simulink subsystem "OGBMS"  (R2020b)
settings: Solver=VariableStepAuto  StartTime=0.0  StopTime=10.0  RelTol=1e-3
libraries: fl_lib x26, nesl_utility x14
settings Model: Creator=marti  LastModifiedBy=MSI PC

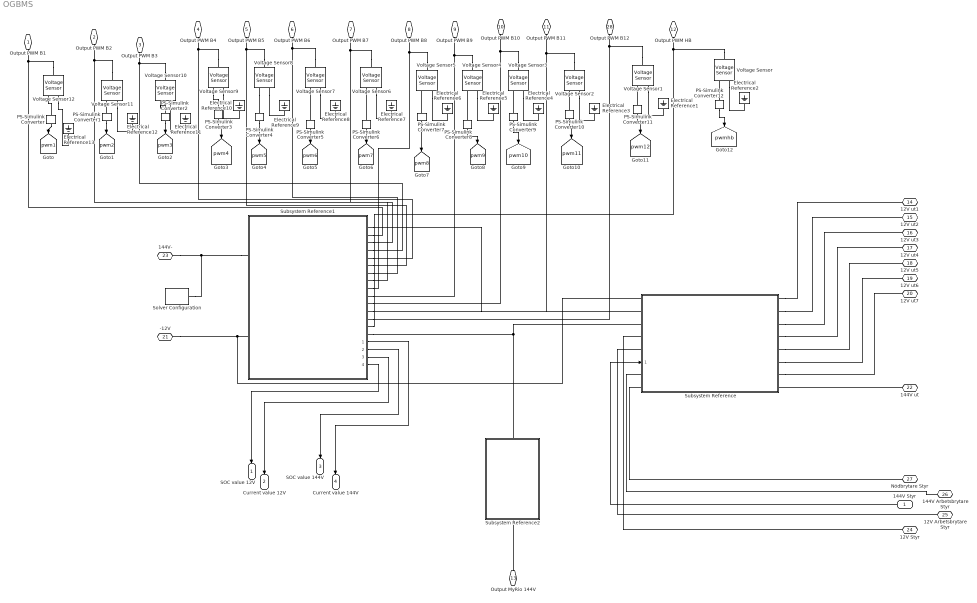
== system OGBMS ==
  144V Styr : Inport
  Electrical Reference{1..13} (13 alike) : fl_lib/Electrical/Electrical Elements/Electrical Reference
  PS-Simulink Converter{,1..12} (13 alike) : nesl_utility/PS-Simulink Converter  PhysicalDomain=network_engine_domain  SubClassName=ps_output  LeftPortType=input  RightPortType=output  PseudoPeriodic=off  Frequencies=[]  Unit=inherit  AffineConversion=off
  Solver Configuration : nesl_utility/Solver Configuration  PhysicalDomain=network_engine_domain  SubClassName=solver  LeftPortType=input  RightPortType=generic  Tones=[]  Harmonics=[]  SimulateNoise=off  Profile=off  UseLocalSampling=off  EnableSwitchedLinearOptims=on  FrequencyDomain=off  UseCCode=off  RelTol=0.001  AbsTol=1e-06  MinStep=1e-09  ToWorkspace=off  RevertToSquareIcSolve=off  NumHomotopyIterations=100  PhasorMode=off  PhasorModeNumHarmonics=1  DoDC=off  ResidualTolerance=1e-09  UseLocalSolver=on  LocalSolverChoice=NE_BACKWARD_EULER_ADVANCER  LocalSolverSampleTime=1e-3  DoFixedCost=on  MaxNonlinIter=3  MaxModeIter=2  ComputeImpulses=off  ImpulseIterations=2  LinearAlgebra=auto  EquationFormulation=NE_TIME_EF  DelaysMemoryBudget=1024  AutomaticFiltering=on  FilteringTimeConstant=0.001  PartitionStorageMethod=AS_NEEDED  PartitionMemoryBudget=1024  PartitionMethod=ROBUST
  Subsystem Reference : Subsystem  ReferencedSubsystem=Brytarsystem_Precharge
      settings: PortSchema="{\"entries\":[{\"content\":{\"sides\":[{\"content\":{\"connectorIds\":[\"LConn2\",\"LConn1\",\"LConn3\",\"LConn4\",\"LConn5\",\"In1\",\"LConn6\",\"LConn7\"]},\"type\":\"ConnectorPlacement.EquallySpacedRectSide\",\"uuid\":\"2795999f-7b79-4b17-9b3a-6c4a2530e28e\"},{\"content\":{\"connectorIds\":[\"RConn1\",\"RConn2\",\"RConn3\",\"RConn4\",\"RConn5\",\"RConn6\",\"RConn7\",\"RConn8\"],\"side\":\"RIGHT\"},\"type\":\"ConnectorPlacement.EquallySpacedRectSide\",\"uuid\":\"43c2790f-657b-4392-8263-a1596afb59fc\"},{\"content\":{\"connectorIds\":[],\"side\":\"TOP\"},\"type\":\"ConnectorPlacement.EquallySpacedRectSide\",\"uuid\":\"569c6d6e-2155-4041-b6f4-fef8df6b1fab\"},{\"content\":{\"connectorIds\":[],\"side\":\"HIDDEN\"},\"type\":\"ConnectorPlacement.EquallySpacedRectSide\",\"uuid\":\"67c7fe8b-d93f-47b6-929e-10fa5a25f6ec\"}]},\"type\":\"ConnectorPlacement.EquallySpacedConnector\",\"uuid\":\"ebaadd78-e701-422e-bc35-4de184f449aa\"}],\"packageUris\":[\"http://schema.mathworks.com/mf0/Connector/R2020b\"],\"version\":\"1.0\"}"
  Subsystem Reference1 : Subsystem  ReferencedSubsystem=Batteri
      settings: PortSchema="{\"entries\":[{\"content\":{\"sides\":[{\"content\":{\"connectorIds\":[\"LConn1\",\"LConn2\"]},\"type\":\"ConnectorPlacement.EquallySpacedRectSide\",\"uuid\":\"b63a6238-416f-4ff8-868a-b1f4009616a2\"},{\"content\":{\"connectorIds\":[\"RConn2\",\"RConn3\",\"RConn4\",\"RConn5\",\"RConn6\",\"RConn7\",\"RConn8\",\"RConn9\",\"RConn10\",\"RConn11\",\"RConn12\",\"RConn13\",\"RConn15\",\"RConn14\",\"RConn1\",\"Out1\",\"Out2\",\"Out3\",\"Out4\"],\"side\":\"RIGHT\"},\"type\":\"ConnectorPlacement.EquallySpacedRectSide\",\"uuid\":\"6b311451-8637-45bf-8d66-5368c1ab9f1f\"},{\"content\":{\"connectorIds\":[],\"side\":\"TOP\"},\"type\":\"ConnectorPlacement.EquallySpacedRectSide\",\"uuid\":\"201ea097-38d5-494b-b753-7ff6c8bbce36\"},{\"content\":{\"connectorIds\":[],\"side\":\"HIDDEN\"},\"type\":\"ConnectorPlacement.EquallySpacedRectSide\",\"uuid\":\"09dcb5d0-90b8-42e6-abba-fd1422207209\"}]},\"type\":\"ConnectorPlacement.EquallySpacedConnector\",\"uuid\":\"e0257631-8d9b-4437-b2cd-348017ba91ab\"}],\"packageUris\":[\"http://schema.mathworks.com/mf0/Connector/R2020b\"],\"version\":\"1.0\"}"
  Subsystem Reference2 : Subsystem  ReferencedSubsystem=Spanningsensor_subsystem
      settings: PortSchema="{\"entries\":[{\"content\":{\"sides\":[{\"content\":{\"connectorIds\":[\"LConn1\"]},\"type\":\"ConnectorPlacement.EquallySpacedRectSide\",\"uuid\":\"e696623b-b3d7-4a4e-997e-08418fead735\"},{\"content\":{\"connectorIds\":[\"LConn2\"],\"side\":\"RIGHT\"},\"type\":\"ConnectorPlacement.EquallySpacedRectSide\",\"uuid\":\"e74a2bad-03ef-4a66-afc0-404d2fc5916d\"},{\"content\":{\"connectorIds\":[],\"side\":\"TOP\"},\"type\":\"ConnectorPlacement.EquallySpacedRectSide\",\"uuid\":\"0eae992c-c63b-47fc-bc32-831da702621f\"},{\"content\":{\"connectorIds\":[],\"side\":\"HIDDEN\"},\"type\":\"ConnectorPlacement.EquallySpacedRectSide\",\"uuid\":\"57c6ecc8-35a0-493f-add2-0a41864266cd\"}]},\"type\":\"ConnectorPlacement.EquallySpacedConnector\",\"uuid\":\"69fce2db-b713-455b-b994-b0b9737411ed\"}],\"packageUris\":[\"http://schema.mathworks.com/mf0/Connector/R2020b\"],\"version\":\"1.0\"}"
  Voltage Sensor{,1..12} (13 alike) : fl_lib/Electrical/Electrical Sensors/Voltage Sensor
  Output PWM B1 : PMIOPort  Side=Left
  Output PWM B2 : PMIOPort  Port=2  Side=Left
  Output PWM B3 : PMIOPort  Port=3  Side=Left
  Output PWM B4 : PMIOPort  Port=4  Side=Left
  Output PWM B5 : PMIOPort  Port=5  Side=Left
  Output PWM B6 : PMIOPort  Port=6  Side=Left
  Output PWM B7 : PMIOPort  Port=7  Side=Left
  Output PWM B8 : PMIOPort  Port=8  Side=Left
  Output PWM B9 : PMIOPort  Port=9  Side=Left
  Output PWM B10 : PMIOPort  Port=10  Side=Left
  Output PWM B11 : PMIOPort  Port=11  Side=Left
  Output PWM HB : PMIOPort  Port=12  Side=Left
  Output MyRio 144V : PMIOPort  Port=13  Side=Left
  12V ut1 : PMIOPort  Port=14  Side=Right
  12V ut2 : PMIOPort  Port=15  Side=Right
  12V ut3 : PMIOPort  Port=16  Side=Right
  12V ut4 : PMIOPort  Port=17  Side=Right
  12V ut5 : PMIOPort  Port=18  Side=Right
  12V ut6 : PMIOPort  Port=19  Side=Right
  12V ut7 : PMIOPort  Port=20  Side=Right
  -12V : PMIOPort  Port=21  Side=Right
  144V ut : PMIOPort  Port=22  Side=Right
  144V- : PMIOPort  Port=23  Side=Right
  "12V Styr " : PMIOPort  Port=24  Side=Right
  12V Arbetsbrytare Styr : PMIOPort  Port=25  Side=Right
  144V Arbetsbrytare Styr : PMIOPort  Port=26  Side=Right
  Nödbrytare Styr : PMIOPort  Port=27  Side=Right
  Output PWM B12 : PMIOPort  Port=28  Side=Left
  SOC value 12V : Outport
  Current value 12V : Outport  Port=2
  SOC value 144V : Outport  Port=3
  Current value 144V : Outport  Port=4
  tag scope: pwm10=global, pwm11=global, pwm12=global, pwm1=global, pwm2=global, pwm3=global, pwm4=global, pwm5=global, pwm6=global, pwm7=global, pwm8=global, pwm9=global, pwmhb=global
  wires:
  Subsystem Reference1/4 -> SOC value 12V/1
  144V Styr/1 -> Subsystem Reference/1
  Subsystem Reference1/1 -> Current value 144V/1
  Subsystem Reference1/3 -> Current value 12V/1
  Subsystem Reference1/2 -> SOC value 144V/1
  PS-Simulink Converter1/1 -> [pwm2]
  PS-Simulink Converter2/1 -> [pwm3]
  PS-Simulink Converter3/1 -> [pwm4]
  PS-Simulink Converter5/1 -> [pwm6]
  PS-Simulink Converter6/1 -> [pwm7]
  PS-Simulink Converter7/1 -> [pwm8]
  PS-Simulink Converter9/1 -> [pwm10]
  PS-Simulink Converter10/1 -> [pwm11]
  PS-Simulink Converter11/1 -> [pwm12]
  PS-Simulink Converter12/1 -> [pwmhb]
  PS-Simulink Converter8/1 -> [pwm9]
  PS-Simulink Converter4/1 -> [pwm5]
  PS-Simulink Converter/1 -> [pwm1]
  connections:
  Subsystem Reference1/LConn1 -- 144V-/RConn1 -- Solver Configuration/RConn1
  Subsystem Reference/LConn2 -- -12V/RConn1 -- Subsystem Reference1/LConn2
  Subsystem Reference1/RConn1 -- Subsystem Reference/LConn3 -- Subsystem Reference2/LConn1
  Voltage Sensor2/LConn1 -- Subsystem Reference1/RConn13 -- Output PWM B11/RConn1
  Voltage Sensor5/LConn1 -- Subsystem Reference1/RConn10 -- Output PWM B8/RConn1
  Voltage Sensor4/LConn1 -- Subsystem Reference1/RConn11 -- Output PWM B9/RConn1
  Voltage Sensor11/LConn1 -- Subsystem Reference1/RConn4 -- Output PWM B2/RConn1
  Voltage Sensor/LConn1 -- Subsystem Reference1/RConn14 -- Output PWM HB/RConn1
  Voltage Sensor12/LConn1 -- Subsystem Reference1/RConn3 -- Output PWM B1/RConn1
  Voltage Sensor6/LConn1 -- Subsystem Reference1/RConn9 -- Output PWM B7/RConn1
  Voltage Sensor9/LConn1 -- Subsystem Reference1/RConn6 -- Output PWM B4/RConn1
  Voltage Sensor3/LConn1 -- Subsystem Reference1/RConn12 -- Output PWM B10/RConn1
  Voltage Sensor10/LConn1 -- Subsystem Reference1/RConn5 -- Output PWM B3/RConn1
  Voltage Sensor7/LConn1 -- Subsystem Reference1/RConn8 -- Output PWM B6/RConn1
  Voltage Sensor8/LConn1 -- Subsystem Reference1/RConn7 -- Output PWM B5/RConn1
  Voltage Sensor1/LConn1 -- Subsystem Reference1/RConn15 -- Output PWM B12/RConn1
  Subsystem Reference/RConn2 -- 12V ut2/RConn1
  Subsystem Reference/RConn1 -- 12V ut1/RConn1
  Subsystem Reference/RConn7 -- 12V ut7/RConn1
  144V ut/RConn1 -- Subsystem Reference/RConn8
  Subsystem Reference/LConn6 -- 144V Arbetsbrytare Styr/RConn1
  Subsystem Reference/LConn7 -- Nödbrytare Styr/RConn1
  12V Arbetsbrytare Styr/RConn1 -- Subsystem Reference/LConn5
  Subsystem Reference/RConn3 -- 12V ut3/RConn1
  Output MyRio 144V/RConn1 -- Subsystem Reference2/LConn2
  Subsystem Reference/RConn4 -- 12V ut4/RConn1
  Subsystem Reference/RConn5 -- 12V ut5/RConn1
  Subsystem Reference1/RConn2 -- Subsystem Reference/LConn1
  Subsystem Reference/RConn6 -- 12V ut6/RConn1
  Subsystem Reference/LConn4 -- "12V Styr "/RConn1
  Voltage Sensor/RConn2 -- Electrical Reference2/LConn1
  Voltage Sensor1/RConn2 -- Electrical Reference1/LConn1
  Voltage Sensor2/RConn2 -- Electrical Reference3/LConn1
  Voltage Sensor3/RConn2 -- Electrical Reference4/LConn1
  Voltage Sensor4/RConn2 -- Electrical Reference5/LConn1
  Voltage Sensor5/RConn2 -- Electrical Reference6/LConn1
  Voltage Sensor6/RConn2 -- Electrical Reference7/LConn1
  Voltage Sensor7/RConn2 -- Electrical Reference8/LConn1
  Voltage Sensor8/RConn2 -- Electrical Reference9/LConn1
  Voltage Sensor9/RConn2 -- Electrical Reference10/LConn1
  Voltage Sensor10/RConn2 -- Electrical Reference11/LConn1
  Voltage Sensor11/RConn2 -- Electrical Reference12/LConn1
  Voltage Sensor12/RConn2 -- Electrical Reference13/LConn1
  PS-Simulink Converter1/LConn1 -- Voltage Sensor11/RConn1
  PS-Simulink Converter5/LConn1 -- Voltage Sensor7/RConn1
  PS-Simulink Converter6/LConn1 -- Voltage Sensor6/RConn1
  PS-Simulink Converter7/LConn1 -- Voltage Sensor5/RConn1
  PS-Simulink Converter8/LConn1 -- Voltage Sensor4/RConn1
  PS-Simulink Converter9/LConn1 -- Voltage Sensor3/RConn1
  PS-Simulink Converter10/LConn1 -- Voltage Sensor2/RConn1
  PS-Simulink Converter11/LConn1 -- Voltage Sensor1/RConn1
  PS-Simulink Converter12/LConn1 -- Voltage Sensor/RConn1
  Voltage Sensor8/RConn1 -- PS-Simulink Converter4/LConn1
  Voltage Sensor9/RConn1 -- PS-Simulink Converter3/LConn1
  Voltage Sensor10/RConn1 -- PS-Simulink Converter2/LConn1
  Voltage Sensor12/RConn1 -- PS-Simulink Converter/LConn1
